simulink model "me312_homework_6"  (R2020b)
settings: Solver=VariableStepAuto  StartTime=0.0  StopTime=10.0  RelTol=1e-3
settings Model: Creator=alant  LastModifiedBy=alant

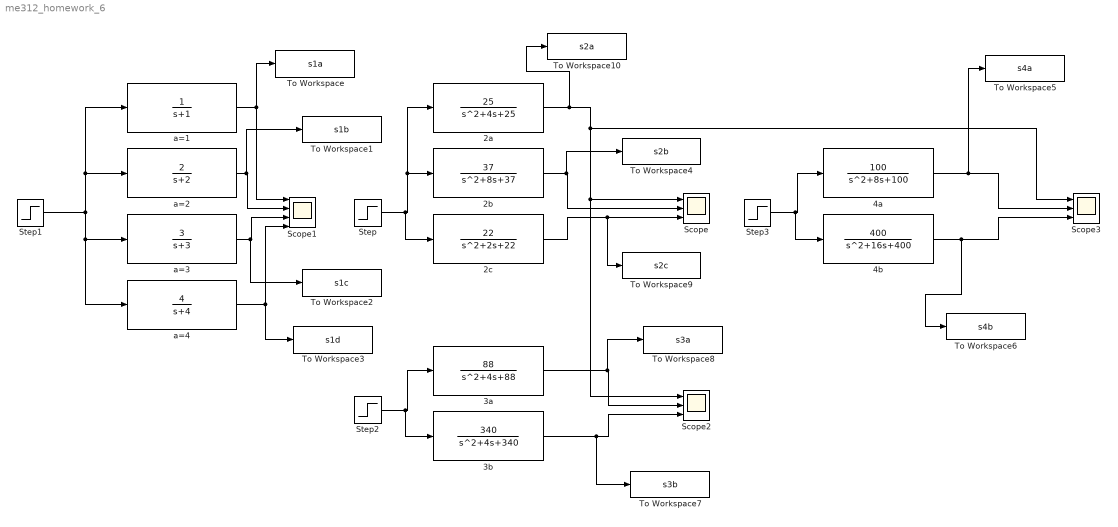
== system me312_homework_6 ==
  2a : TransferFcn  Numerator=25  Denominator=[1 4 25]
  2b : TransferFcn  Numerator=37  Denominator=[1 8 37]
  2c : TransferFcn  Numerator=22  Denominator=[1 2 22]
  3a : TransferFcn  Numerator=88  Denominator=[1 4 88]
  3b : TransferFcn  Numerator=340  Denominator=[1 4 340]
  4a : TransferFcn  Numerator=100  Denominator=[1 8 100]
  4b : TransferFcn  Numerator=400  Denominator=[1 16 400]
  Scope : Scope  NumInputPorts=3
  Scope1 : Scope  NumInputPorts=4
  Scope2 : Scope  NumInputPorts=3
  Scope3 : Scope  NumInputPorts=3
  Step{,1..3} (4 alike) : Step  SampleTime=0
  To Workspace : ToWorkspace  VariableName=s1a  SampleTime=-1
  To Workspace1 : ToWorkspace  VariableName=s1b  SampleTime=-1
  To Workspace10 : ToWorkspace  VariableName=s2a  SampleTime=-1
  To Workspace2 : ToWorkspace  VariableName=s1c  SampleTime=-1
  To Workspace3 : ToWorkspace  VariableName=s1d  SampleTime=-1
  To Workspace4 : ToWorkspace  VariableName=s2b  SampleTime=-1
  To Workspace5 : ToWorkspace  VariableName=s4a  SampleTime=-1
  To Workspace6 : ToWorkspace  VariableName=s4b  SampleTime=-1
  To Workspace7 : ToWorkspace  VariableName=s3b  SampleTime=-1
  To Workspace8 : ToWorkspace  VariableName=s3a  SampleTime=-1
  To Workspace9 : ToWorkspace  VariableName=s2c  SampleTime=-1
  a=1 : TransferFcn  Numerator=1  Denominator=[1 1]
  a=2 : TransferFcn  Numerator=2  Denominator=[1 2]
  a=3 : TransferFcn  Numerator=3  Denominator=[1 3]
  a=4 : TransferFcn  Numerator=4  Denominator=[1 4]
  wires:
  2b/1 -> To Workspace4/1, Scope/2
  2c/1 -> To Workspace9/1, Scope/3
  Step/1 -> 2c/1, 2b/1, 2a/1
  a=3/1 -> To Workspace2/1, Scope1/3
  a=2/1 -> To Workspace1/1, Scope1/2
  a=4/1 -> To Workspace3/1, Scope1/4
  Step1/1 -> a=2/1, a=1/1, a=3/1, a=4/1
  3b/1 -> To Workspace7/1, Scope2/3
  3a/1 -> To Workspace8/1, Scope2/2
  Step2/1 -> 3b/1, 3a/1
  4b/1 -> To Workspace6/1, Scope3/3
  4a/1 -> To Workspace5/1, Scope3/2
  Step3/1 -> 4b/1, 4a/1
  2a/1 -> To Workspace10/1, Scope3/1, Scope2/1, Scope/1
  a=1/1 -> Scope1/1, To Workspace/1
